simulink model "m705"  (Simulink 6.1)
settings: Solver=ode45  StartTime=0.0  StopTime=10.0  RelTol=1e-3
settings Model: LastModifiedBy=okawa
settings DebuggingCC: SolverPrmCheckMsg=warning

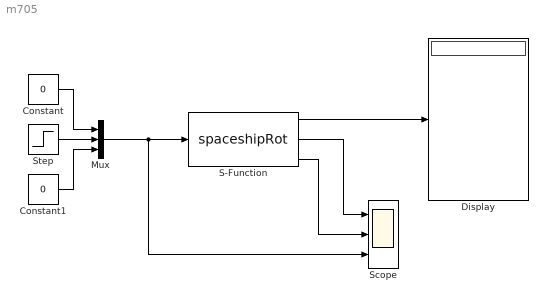
== system m705 ==
  Constant : Constant  Value=0
  Constant1 : Constant  Value=0
  Display : Display
  Mux : Mux  Inputs=3
  S-Function : S-Function  FunctionName=spaceshipRot
  Scope : Scope  NumInputPorts=3
      settings: YMin=-5~-5~-5  YMax=5~5~5
  Step : Step  SampleTime=0
  wires:
  Constant/1 -> Mux/1
  Step/1 -> Mux/2
  Constant1/1 -> Mux/3
  Mux/1 -> S-Function/1, Scope/3
  S-Function/1 -> Display/1
  S-Function/2 -> Scope/1
  S-Function/3 -> Scope/2
